simulink model "sine_9sugeno_wtsum_nothing"  (R2017b)
settings: Solver=FixedStepAuto  StartTime=0.0  StopTime=500.0  RelTol=1e-3  EnableMultiTasking=on
libraries: fuzblock x1
settings Model: Creator=metalhead  LastModifiedBy=root
settings DataIOCC: LimitDataPoints=on
settings OptimizationCC: LifeSpan=inf
settings DebuggingCC: AllowSymbolicDim=off  SFUnexpectedBacktrackingDiag=warning  SFNoUnconditionalDefaultTransitionDiag=warning  SFExecutionAtInitializationDiag=none
settings ModelReferenceCC: PropagateSignalLabelsOutOfModel=off
settings CodeAppCC: StateflowObjectComments=on
settings GRTTargetCC: TargetLangStandard=C89/C90 (ANSI)
settings ConfigComp: CovMetricSettings=dw  CovHtmlReporting=on  CovSaveCumulativeToWorkspaceVar=on  CovSaveSingleToWorkspaceVar=on  CovExternalEMLEnable=off

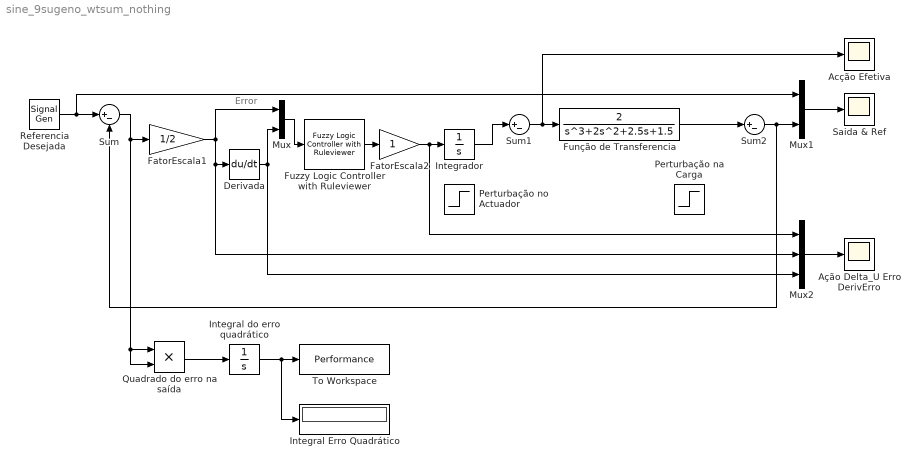
== system sine_9sugeno_wtsum_nothing ==
  note: Error
  Acção Efetiva : Scope
  Ação Delta_U Erro DerivErro : Scope
  Derivada : Derivative
  FatorEscala1 : Gain  Gain=1/2
  FatorEscala2 : Gain
  Função de Transferencia : TransferFcn  Numerator=[2]  Denominator=[1 2 2.5 1.5]
  Fuzzy Logic Controller with Ruleviewer : fuzblock/Fuzzy Logic  Controller  with Ruleviewer  fismatrix=controller11  Ts=1
  Integrador : Integrator
  Integral Erro Quadrático : Display
  Integral do erro quadrático : Integrator
  Mux : Mux  Inputs=2
  Mux1 : Mux  Inputs=2
  Mux2 : Mux  Inputs=3
  Perturbação na Carga : Step  Time=100  SampleTime=0
  Perturbação no Actuador : Step  Time=100  SampleTime=0
  Quadrado do erro na saída : Product
  "Referencia Desejada " : SignalGenerator  Amplitude=-1  Frequency=0.01  Units=rad/sec
  Saida & Ref : Scope
  Sum : Sum  Inputs=|+-
  Sum1 : Sum  Inputs=|+-
  Sum2 : Sum  Inputs=|+-
  To Workspace : ToWorkspace  VariableName=Performance  SaveFormat=Timeseries  SampleTime=-1
  wires:
  "Referencia Desejada "/1 -> Mux1/1, Sum/1
  Sum/1 -> Quadrado do erro na saída/2, Quadrado do erro na saída/1, FatorEscala1/1
  Derivada/1 -> Mux2/3, Mux/2
  FatorEscala1/1 -> Mux/1, Mux2/2, Derivada/1
  FatorEscala2/1 -> Mux2/1, Integrador/1
  Integrador/1 -> Sum1/1
  Sum1/1 -> Acção Efetiva/1, Função de Transferencia/1
  Função de Transferencia/1 -> Sum2/1
  Sum2/1 -> Sum/2, Mux1/2
  Mux1/1 -> Saida & Ref/1
  Mux2/1 -> Ação Delta_U Erro DerivErro/1
  Quadrado do erro na saída/1 -> Integral do erro quadrático/1
  Integral do erro quadrático/1 -> Integral Erro Quadrático/1, To Workspace/1
  Fuzzy Logic Controller with Ruleviewer/1 -> FatorEscala2/1
  Mux/1 -> Fuzzy Logic Controller with Ruleviewer/1
